simulink model "astron_hw_test_skarab_16k"  (R2021a)
settings: Solver=VariableStepDiscrete  StartTime=0.0  StopTime=sim_len  RelTol=1e-3
undefined symbols (not defined in the file): d0, d1, d2, d3, FFT, sr, Wideband_FFT
libraries: xbsIndex_r4 x895, casper_library_misc x4, xps_library x1
(part 5 of 16)

== system astron_hw_test_skarab_16k/bram_in2 ==
  addr : Inport
  data_in : Inport  Port=2
  we : Inport  Port=3
  Terminator : Terminator
  Terminator1 : Terminator
  Terminator2 : Terminator
  astron_hw_test_skarab_16k_bram_in2_addr : xbsIndex_r4/Gateway Out  inherit_from_input=off  hdl_port=on  rows=1  columns=1  UseAsDAC=off  DACChannel='1'  interface=None  automatic_assignment=on  address_offset=hex2dec('00')  intf_name=''  intf_description=''  timing_constraint=None  locs_specified=off  LOCs={'A5','B9','A9','C1','A3','G6','E9','A6','A7','A8','B8','B1','B3','D9','B5','B4','B6','C2'}  io_standard={}  block_type=gatewayout
      settings: infoedit="Gateway out block.  Converts Xilinx fixed point inputs into ouputs of type Simulink integer, double, or fixed point.<P><P>Hardware notes:  In hardware these blocks become top level output ports or are discarded, depending on how they are configured."  sginterface={'Nallatech'=>{'xdspkit'=>{'non_memory_mapped_port'=>'uprev_Shared_BRAM_addr'}},'Xilinx'=>{'jtaghwcosim'=>{'non_memory_mapped_port'=>'uprev_Shared_BRAM_addr'},'xdspkit'=>{'non_memory_mapped_port'=>'uprev_Shared_BRAM_addr'}}}  xl_area=[0, 0, 0, 0, 0, 0, 0]
  astron_hw_test_skarab_16k_bram_in2_data_in : xbsIndex_r4/Gateway Out  inherit_from_input=off  hdl_port=on  rows=1  columns=1  UseAsDAC=off  DACChannel='1'  interface=None  automatic_assignment=on  address_offset=hex2dec('00')  intf_name=''  intf_description=''  timing_constraint=None  locs_specified=off  LOCs={'B21','B22','A22','B23','B19','C19','A20','A21','A23','B24','A24','A25','E18','D18','C18','B18'}  io_standard={}  block_type=gatewayout
      settings: infoedit="Gateway out block.  Converts Xilinx fixed point inputs into ouputs of type Simulink integer, double, or fixed point.<P><P>Hardware notes:  In hardware these blocks become top level output ports or are discarded, depending on how they are configured."  sginterface={'Nallatech'=>{'xdspkit'=>{'non_memory_mapped_port'=>'uprev_Shared_BRAM_data_in'}},'Xilinx'=>{'jtaghwcosim'=>{'non_memory_mapped_port'=>'uprev_Shared_BRAM_data_in'},'xdspkit'=>{'non_memory_mapped_port'=>'uprev_Shared_BRAM_data_in'}}}  xl_area=[0, 0, 0, 0, 0, 0, 0]
  astron_hw_test_skarab_16k_bram_in2_data_out : xbsIndex_r4/Gateway In  gui_display_data_type=Fixed-point  arith_type=Unsigned  n_bits=32  bin_pt=0  preci_type=Single  exp_width=8  frac_width=24  rows=1  columns=1  quantization=Truncate  overflow=Wrap  period=sample_rate  UseAsADC=off  ADCChannel='1'  interface=None  automatic_assignment=on  address_offset=hex2dec('00')  intf_name=''  intf_description=''  default_value=0  timing_constraint=None  locs_specified=off  LOCs={}  io_standard={}  inherit_from_input=off  hdl_port=on  dbl_ovrd=off  block_type=gatewayin
      settings: xl_area=[0, 0, 0, 0, 0, 0, 0]
  astron_hw_test_skarab_16k_bram_in2_we : xbsIndex_r4/Gateway Out  inherit_from_input=off  hdl_port=on  rows=1  columns=1  UseAsDAC=off  DACChannel='1'  interface=None  automatic_assignment=on  address_offset=hex2dec('00')  intf_name=''  intf_description=''  timing_constraint=None  locs_specified=off  LOCs={'A14'}  io_standard={}  block_type=gatewayout
      settings: infoedit="Gateway out block.  Converts Xilinx fixed point inputs into ouputs of type Simulink integer, double, or fixed point.<P><P>Hardware notes:  In hardware these blocks become top level output ports or are discarded, depending on how they are configured."  xl_area=[0, 0, 0, 0, 0, 0, 0]
  calc_add : Subsystem  mask{data_width=32, addr_width=12, sample_rate=sample_rate}
      mask prompts: data_width "data width"; addr_width "address width"; sample_rate "sample rate"
  convert_addr : xbsIndex_r4/Convert  gui_display_data_type=Fixed-point  arith_type=Unsigned  n_bits=addr_width  bin_pt=0  float_type=Single  exp_bits=8  fraction_bits=24  quantization=Truncate  overflow=Wrap  en=off  latency=0  pipeline=off  dbl_ovrd=off  block_type=convert
      settings: xl_area=[0, 0, 0, 0, 0, 0, 0]
  convert_din1 : xbsIndex_r4/Convert  gui_display_data_type=Fixed-point  arith_type=Unsigned  n_bits=32  bin_pt=0  float_type=Single  exp_bits=8  fraction_bits=24  quantization=Truncate  overflow=Wrap  en=off  latency=0  pipeline=off  dbl_ovrd=off  block_type=convert
      settings: xl_area=[0, 0, 0, 0, 0, 0, 0]
  convert_we : xbsIndex_r4/Convert  gui_display_data_type=Fixed-point  arith_type=Unsigned  n_bits=1  bin_pt=0  float_type=Single  exp_bits=8  fraction_bits=24  quantization=Truncate  overflow=Wrap  en=off  latency=0  pipeline=off  dbl_ovrd=off  block_type=convert
      settings: xl_area=[0, 0, 0, 0, 0, 0, 0]
  munge_in : Subsystem  AncestorBlock=casper_library_flow_control/munge  mask(munge){divisions=1, div_size=32, order=[0], arith_type_out=Unsigned, bin_pt_out=0}
      mask prompts: divisions "Number of divisions"; div_size "Division size (bits)"; order "Division packing order"; arith_type_out "Output arithmetic type"; bin_pt_out "Output binary point"
      mask help: Splits an input bus into the specified number of divisions and then recombines them in the order specified (most significant division = 0,least = number divisions-1)
      mask init:
      | munge_init(gcb, ...
      |     'divisions', divisions, ...
      |     'div_size', div_size, ...
      |     'order', order, ...
      |     'arith_type_out', arith_type_out, ...
      |     'bin_pt_out', bin_pt_out);
      settings: AttributesFormatString=|
      | split:32
      | join:0
      | Unsigned [32,0]
      mask TypeOptions arith_type_out: Unsigned | Signed  (2's comp) | Floating-point
  munge_out : Subsystem  AncestorBlock=casper_library_flow_control/munge  mask(munge){divisions=1, div_size=32, order=[0], arith_type_out=Signed  (2's comp), bin_pt_out=0}
      mask prompts: divisions "Number of divisions"; div_size "Division size (bits)"; order "Division packing order"; arith_type_out "Output arithmetic type"; bin_pt_out "Output binary point"
      mask help: Splits an input bus into the specified number of divisions and then recombines them in the order specified (most significant division = 0,least = number divisions-1)
      mask init:
      | munge_init(gcb, ...
      |     'divisions', divisions, ...
      |     'div_size', div_size, ...
      |     'order', order, ...
      |     'arith_type_out', arith_type_out, ...
      |     'bin_pt_out', bin_pt_out);
      settings: AttributesFormatString=|
      | split:32
      | join:0
      | Signed  (2's comp) [32,0]
      mask TypeOptions arith_type_out: Unsigned | Signed  (2's comp) | Floating-point
  sim_mem : Subsystem  mask{arith_type=Signed  (2's comp), addr_width=12, data_width=32, data_bin_pt=0, init_vals=[-2187   5793  -5143  -1458   2477   4757  -4236   1335  -1089  -2579  -2505   6267    423  -4130  -2579   5928  -3270   5563  -1943  -7422  -2024   -739  -3142  -1014   5972   1714  -1074   1726   1567     95  -6816   -238  -1787   8345   -609   3629  11789  -1835   1592   3599  -1729  -3355  -1269  -8095  -2092  10467  -2924  -2289   4751   4898   1360    711   7466   1068   3501  -3077   6185   -699  -7850   1750  -1330  -4192    -64   2955    580   6927   1217  -1648   3895    786   2361   2632  -5762   -836  -3707   5736   5110   1213  -4438  -3757   1834   2783  -2890    579     90   6274   3034  -6269    856   -321   5267  -1127   3973   8055  -5345   1612   5672  -5108   8343   5006  -3883   2466  -4226   1404   1310   1625  -9157  -4794   4156   3778  -6287  -9301   8373   2006    703  -1493   2358   1477   2560  -1749   2143   1774  -5195    942  -3895   2502  -1517  -6457   5485  -6201   3318     61  -1232  -5876  -1696   1668  -2100   1620    251   -902   1687   4484  -1999 -13066  -1146    754  -1964  -5446   1808   1608   1860  -2616  -4527  -4606  -2881   4527   3649   4601   4127  -2884  12407   9028   2401  -3584   -169   3461   7313  -3652  -1293   2359    -66   -738  -1895   9008  -5249  -4845   -237  -3879  -1188   2315   1725  -1416    261   2197  -5363   1295   1305  -9118   6011   4545   -163   3868   3357   9920   1846 -10434   -719   2524  -4826   1766    746  -7716  -2627   8394  -2322  -6696   2881   2124  -6395   6728  -6941   2027   -242  -2604     81  -1058   3227    392  -8820   2434  12584  -6210  -4059    -90   2619   1863    159   2515   1125  -4145  -5260   4722   3343   -309  -3657  -1534   1602   -410  -1519   -937    -92   1026   1374   5505   -561  -3172   -983  -1848   2928    -34  -6456  -4085    606   1933  -8205   2778    722   3176  -1470  -3061   2024   1535  -4073  -7446   4633  10816  -1566  -3810   3543   3442  -1765   4846  -2996   3576   3364  -8299  -1533  -6720   3600  -6133   5687  -5295  -4130  -1533  -5778   -332   3425  -6125   3075   1895  -3860  -7377   1343   -854  -2825 -13842   1499  -2746   -134  -1496   3651  -3121  -3432  -4217  -1491   -418  -4742  -3629   5015   6034   2283  -5871  -1666   3414  -5499   1724   4075  -2000  -4226   3516   3290   6703   5505    807  -5100    949   3489   3303  -1818   7784  -5453   3579   9662   5374   2006   1128   9584    611   1526   2509  -1416  -2470   6707   -276   2613  -2156    -69   7215   1180     83   -719  -1295   5837   4694  -1311  -1272    922   2409 -10814   -354  -2707    -35   2796  -1072   6387   2062   1555  -1304    169   2287  -6434  -7241  -4654   1632  -7556  -3711  -4949    749  -5218    -73  -2140  12007   7069   -328   8829  -6116  -1706  -4758   2687   5796   3841   2920   1352  -5213    409  -1011  -7232     85  -1245  -3271  -5390   3603  -2129  -1153  -4609   3407    434  -5838   3517   6625 -11826    894  -2405  -2563   2265  -4260   7997  -3703   4596   3724  -7539  -5529  -9153  -2079   -871   2216   -590   -929   2679   3073  -5272  -1164  -2745  -1039  -7273   7827   -420  -3245  -2124  -4949   2455   2454  -4939  -7344   9201   2964   1792  -8513  -5971   2321  -1960   1187  -1488   2078   3236    120   4897   3962  -2597  -2485  -4494  -1035    123     79   1998  -3039   -563 -11520  -1833   1544  -1861   1115   1501   2083  -1650  -3776   6906   1747  -8591  -2639   2565   2572  -3821   6721  -2579  -5558   3938   -629  -1556   -196   -821  -3301   3965   -435   1164  -3604  -1278    987  -2157   4793   8239    454  -3147  -1401  -2274  -4113  -2355  -3505    907   8573  -4974   -703    612   1067  -4420   4250  -7353   2288  -5183    843   3063    844   1351  -9882    247   3231   2291  -4192    363   7850   1281  -3413   2112   5420  -2203    617  -5980   1423  -5088   2354   9044    260   1382  -2229  -3646   5491   -482   4754    151  -1955   1462  -4761     89   1357  -3347   2736  -3864  -4020    314   3685   3845  -5469  -2582   -725   4782   -591  -3114  -6913   5829   4729    409 ...(+24674 chars)], sample_rate=1, csp_latency=1}
      mask prompts: arith_type "Output Data Type"; addr_width "Address width"; data_width "Data width"; data_bin_pt "Data Binary Point"; init_vals "Initial values"; sample_rate "Sample rate"; csp_latency "Latency"
      mask init:
      | % set_param([gcb, '/data_to_xilinx'], 'arith_type', arith_type)
      | % set_param([gcb, '/data_to_xilinx'], 'n_bits', get_param(gcb, 'data_width'))
      mask TypeOptions arith_type: Unsigned | Signed  (2's comp)
      mask TypeOptions data_width: 8 | 16 | 32 | 64 | 128
  data_out : Outport  VectorParamsAs1DForOutWhenUnconnected=off
  wires:
  munge_out/1(dout) -> data_out/1
  sim_mem/1(data_out) -> astron_hw_test_skarab_16k_bram_in2_data_out/1
  astron_hw_test_skarab_16k_bram_in2_data_out/1 -> munge_out/1(din)
  convert_addr/1 -> astron_hw_test_skarab_16k_bram_in2_addr/1
  convert_din1/1 -> astron_hw_test_skarab_16k_bram_in2_data_in/1
  data_in/1 -> munge_in/1(din)
  calc_add/1(out) -> convert_addr/1
  astron_hw_test_skarab_16k_bram_in2_we/1 -> Terminator2/1
  astron_hw_test_skarab_16k_bram_in2_data_in/1 -> Terminator1/1
  astron_hw_test_skarab_16k_bram_in2_addr/1 -> Terminator/1
  convert_we/1 -> astron_hw_test_skarab_16k_bram_in2_we/1
  addr/1 -> sim_mem/1(addr), calc_add/1(in)
  we/1 -> sim_mem/3(we), convert_we/1
  munge_in/1(dout) -> sim_mem/2(data), convert_din1/1
